simulink model "LQR_Controller"  (R2023b)
settings: Solver=VariableStepAuto  StartTime=0.0  StopTime=100  RelTol=1e-3
values from neighbouring files (symbols this model uses):
  k1 = K(3,1)    [LQR.m]
  k10 = K(3,10)    [LQR.m]
  k11 = K(4,11)    [LQR.m]
  k12 = K(4,12)    [LQR.m]
  k2 = K(3,2)    [LQR.m]
  k3 = K(2,3)    [LQR.m]
  k5 = K(1,5)    [LQR.m]
  k6 = K(1,6)    [LQR.m]
  k7 = K(2,7)    [LQR.m]
  k8 = K(2,8)    [LQR.m]
  k9 = K(3,9)    [LQR.m]
  ki13 = Ki(3,13)    [LQR.m]
  ki14 = Ki(2,14)    [LQR.m]
undefined symbols (not defined in the file or in its folder): g, m
settings Model: Creator=DELL  LastModifiedBy=DELL

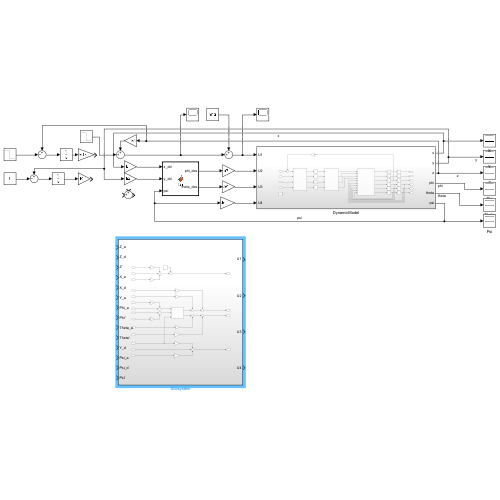
[thumbnail: Simulink's stored preview of the top-level diagram]
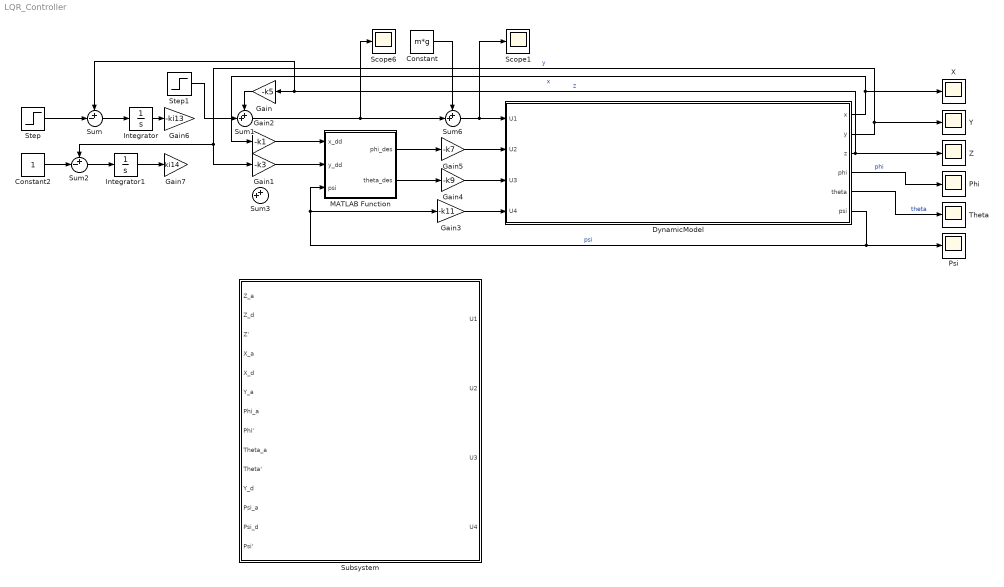
== system LQR_Controller ==
  Constant : Constant  Value=m*g
  Constant2 : Constant
  DynamicModel : Subsystem
  Gain : Gain  Gain=-k5
  Gain1 : Gain  Gain=-k3
  Gain2 : Gain  Gain=-k1
  Gain3 : Gain  Gain=-k11
  Gain4 : Gain  Gain=-k9
  Gain5 : Gain  Gain=-k7
  Gain6 : Gain  Gain=-ki13
  Gain7 : Gain  Gain=ki14
  Integrator : Integrator
  Integrator1 : Integrator
  MATLAB Function : MATLAB Function  TreatAsAtomicUnit=on
  Phi : Scope
  Psi : Scope
  Scope1 : Scope
  Scope6 : Scope
  Step : Step  After=-1  SampleTime=0
  Step1 : Step  After=-1  SampleTime=0
  Subsystem : Subsystem
  Sum : Sum  Inputs=+-|
  Sum1 : Sum  Inputs=++|
  Sum2 : Sum  Inputs=+-|
  Sum3 : Sum  Inputs=++|
  Sum6 : Sum  Inputs=++|
  Theta : Scope
  X : Scope
  Y : Scope
  Z : Scope
  wires:
  DynamicModel/3(z) -> Z/1, Sum/1, Gain/1  "z"
  DynamicModel/2(y) -> Y/1, Sum2/1, Gain1/1  "y"
  DynamicModel/1(x) -> Gain2/1, X/1  "x"
  DynamicModel/6(psi) -> Psi/1, Gain3/1, MATLAB Function/3(psi)  "psi"
  DynamicModel/4(phi) -> Phi/1  "phi"
  DynamicModel/5(theta) -> Theta/1  "theta"
  MATLAB Function/2(theta_des) -> Gain4/1
  Gain2/1 -> MATLAB Function/1(x_dd)
  Gain3/1 -> DynamicModel/4(U4)
  MATLAB Function/1(phi_des) -> Gain5/1
  Gain5/1 -> DynamicModel/2(U2)
  Gain4/1 -> DynamicModel/3(U3)
  Sum6/1 -> Scope1/1, DynamicModel/1(U1)
  Constant/1 -> Sum6/1
  Step/1 -> Sum/2
  Sum/1 -> Integrator/1
  Integrator/1 -> Gain6/1
  Gain/1 -> Sum1/1
  Sum1/1 -> Sum6/2, Scope6/1
  Integrator1/1 -> Gain7/1
  Sum2/1 -> Integrator1/1
  Constant2/1 -> Sum2/2
  Step1/1 -> Sum1/2
  Gain1/1 -> MATLAB Function/2(y_dd)

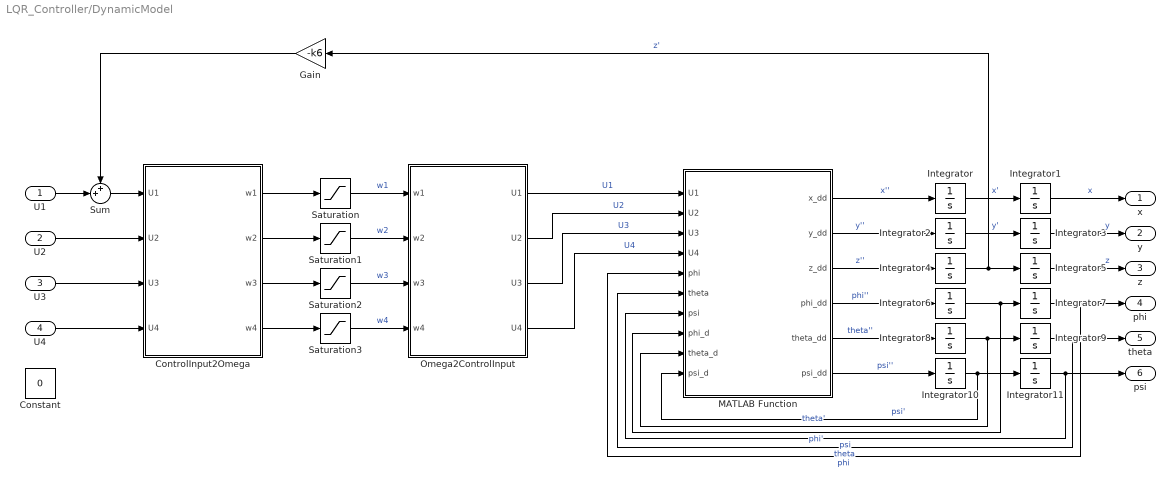
== system LQR_Controller/DynamicModel ==
  U1 : Inport
  U2 : Inport  Port=2
  U3 : Inport  Port=3
  U4 : Inport  Port=4
  Constant : Constant  Value=0
  ControlInput2Omega : MATLAB Function  TreatAsAtomicUnit=on
  Gain : Gain  Gain=-k6
  Integrator{,1..11} (12 alike) : Integrator
  MATLAB Function : MATLAB Function  TreatAsAtomicUnit=on
  Omega2ControlInput : MATLAB Function  TreatAsAtomicUnit=on
  Saturation{,1..3} (4 alike) : Saturate  UpperLimit=550  LowerLimit=0
  Sum : Sum  Inputs=++|
  x : Outport
  y : Outport  Port=2
  z : Outport  Port=3
  phi : Outport  Port=4
  theta : Outport  Port=5
  psi : Outport  Port=6
  wires:
  Integrator8/1 -> MATLAB Function/9(theta_d), Integrator9/1  "theta'"
  ControlInput2Omega/3(w3) -> Saturation2/1
  Integrator5/1 -> z/1  "z"
  MATLAB Function/1(x_dd) -> Integrator/1  "x''"
  MATLAB Function/5(theta_dd) -> Integrator8/1  "theta''"
  MATLAB Function/6(psi_dd) -> Integrator10/1  "psi''"
  MATLAB Function/3(z_dd) -> Integrator4/1  "z''"
  Saturation2/1 -> Omega2ControlInput/3(w3)  "w3"
  Integrator10/1 -> MATLAB Function/10(psi_d), Integrator11/1  "psi'"
  Integrator6/1 -> MATLAB Function/8(phi_d), Integrator7/1  "phi'"
  MATLAB Function/4(phi_dd) -> Integrator6/1  "phi''"
  Integrator3/1 -> y/1  "y"
  Saturation1/1 -> Omega2ControlInput/2(w2)  "w2"
  ControlInput2Omega/4(w4) -> Saturation3/1
  Integrator4/1 -> Gain/1, Integrator5/1  "z'"
  Saturation/1 -> Omega2ControlInput/1(w1)  "w1"
  Saturation3/1 -> Omega2ControlInput/4(w4)  "w4"
  Integrator11/1 -> psi/1, MATLAB Function/7(psi)  "psi"
  MATLAB Function/2(y_dd) -> Integrator2/1  "y''"
  Integrator2/1 -> Integrator3/1  "y'"
  Integrator7/1 -> phi/1, MATLAB Function/5(phi)  "phi"
  Integrator1/1 -> x/1  "x"
  Integrator/1 -> Integrator1/1  "x'"
  ControlInput2Omega/2(w2) -> Saturation1/1
  Integrator9/1 -> theta/1, MATLAB Function/6(theta)  "theta"
  ControlInput2Omega/1(w1) -> Saturation/1
  Omega2ControlInput/1(U1) -> MATLAB Function/1(U1)  "U1"
  Omega2ControlInput/2(U2) -> MATLAB Function/2(U2)  "U2"
  Omega2ControlInput/3(U3) -> MATLAB Function/3(U3)  "U3"
  Omega2ControlInput/4(U4) -> MATLAB Function/4(U4)  "U4"
  U4/1 -> ControlInput2Omega/4(U4)
  U3/1 -> ControlInput2Omega/3(U3)
  U2/1 -> ControlInput2Omega/2(U2)
  U1/1 -> Sum/2
  Sum/1 -> ControlInput2Omega/1(U1)
  Gain/1 -> Sum/1

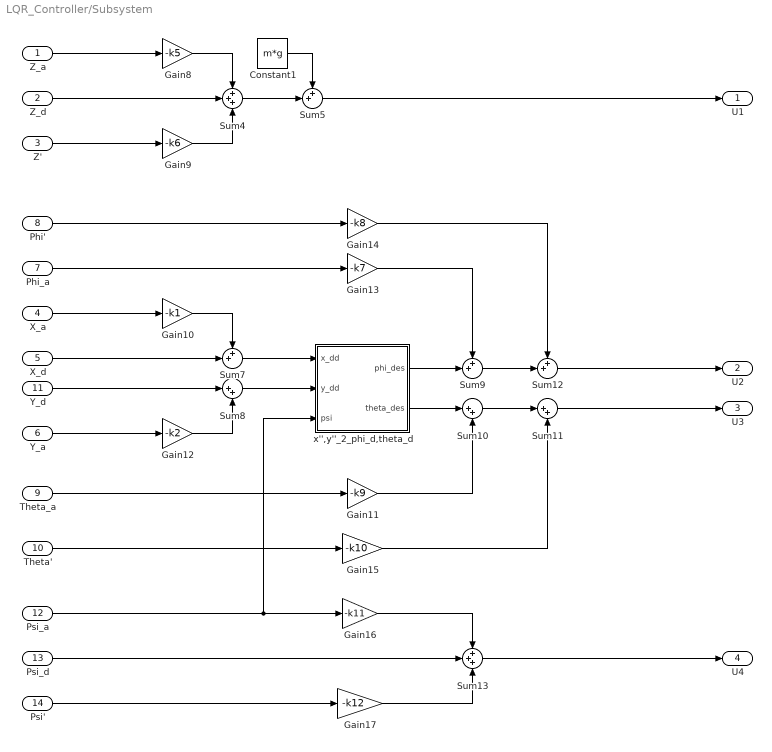
== system LQR_Controller/Subsystem ==
  Z_a : Inport
  Z_d : Inport  Port=2
  Z' : Inport  Port=3
  X_a : Inport  Port=4
  X_d : Inport  Port=5
  Y_a : Inport  Port=6
  Phi_a : Inport  Port=7
  Phi' : Inport  Port=8
  Theta_a : Inport  Port=9
  Theta' : Inport  Port=10
  Y_d : Inport  Port=11
  Psi_a : Inport  Port=12
  Psi_d : Inport  Port=13
  Psi' : Inport  Port=14
  Constant1 : Constant  Value=m*g
  Gain10 : Gain  Gain=-k1
  Gain11 : Gain  Gain=-k9
  Gain12 : Gain  Gain=-k2
  Gain13 : Gain  Gain=-k7
  Gain14 : Gain  Gain=-k8
  Gain15 : Gain  Gain=-k10
  Gain16 : Gain  Gain=-k11
  Gain17 : Gain  Gain=-k12
  Gain8 : Gain  Gain=-k5
  Gain9 : Gain  Gain=-k6
  Sum10 : Sum  Inputs=|++
  Sum11 : Sum  Inputs=|++
  Sum{5,7,9,12} (4 alike) : Sum  Inputs=++|
  Sum13 : Sum  Inputs=+++
  Sum4 : Sum  Inputs=+++
  Sum8 : Sum  Inputs=|++
  x'',y''_2_phi_d,theta_d : MATLAB Function  TreatAsAtomicUnit=on
  U1 : Outport
  U2 : Outport  Port=2
  U3 : Outport  Port=3
  U4 : Outport  Port=4
  wires:
  Theta_a/1 -> Gain11/1
  Gain8/1 -> Sum4/1
  x'',y''_2_phi_d,theta_d/2(theta_des) -> Sum10/1
  X_a/1 -> Gain10/1
  Y_a/1 -> Gain12/1
  Sum12/1 -> U2/1
  Z'/1 -> Gain9/1
  Gain17/1 -> Sum13/3
  Sum13/1 -> U4/1
  X_d/1 -> Sum7/2
  Sum8/1 -> x'',y''_2_phi_d,theta_d/2(y_dd)
  Sum4/1 -> Sum5/2
  Psi'/1 -> Gain17/1
  Z_a/1 -> Gain8/1
  Sum9/1 -> Sum12/2
  Gain9/1 -> Sum4/3
  Phi'/1 -> Gain14/1
  Gain16/1 -> Sum13/1
  Gain15/1 -> Sum11/2
  Y_d/1 -> Sum8/1
  Constant1/1 -> Sum5/1
  Gain13/1 -> Sum9/1
  Phi_a/1 -> Gain13/1
  Gain10/1 -> Sum7/1
  x'',y''_2_phi_d,theta_d/1(phi_des) -> Sum9/2
  Sum7/1 -> x'',y''_2_phi_d,theta_d/1(x_dd)
  Gain12/1 -> Sum8/2
  Gain14/1 -> Sum12/1
  Gain11/1 -> Sum10/2
  Psi_d/1 -> Sum13/2
  Sum10/1 -> Sum11/1
  Psi_a/1 -> x'',y''_2_phi_d,theta_d/3(psi), Gain16/1
  Sum11/1 -> U3/1
  Sum5/1 -> U1/1
  Theta'/1 -> Gain15/1
  Z_d/1 -> Sum4/2

== matlab function LQR_Controller/DynamicModel/Omega2ControlInput ==
  data: w1 input; U1 output; w2 input; w3 input; w4 input; U2 output; U3 output; U4 output
function [U1,U2,U3,U4] = fcn(w1,w2,w3,w4)
    
    % COEFFITIENTS
    Kf = 3.13e-5;
    Km = 7.5e-7;

    U1 = Kf * ((w1^2)+(w2^2)+(w3^2)+(w4^2));
    U2 = Kf * (-(w2^2)+(w4^2));
    U3 = Kf * ((w1^2)-(w3^2));
    U4 = Km * ((w1^2)-(w2^2)+(w3^2)-(w4^2));

== matlab function LQR_Controller/DynamicModel/MATLAB Function ==
  data: U1 input; x_dd output; U2 input; U3 input; U4 input; phi input; theta input; psi input; phi_d input; theta_d input; psi_d input; y_dd output; z_dd output; phi_dd output; theta_dd output; psi_dd output
function [x_dd,y_dd,z_dd,phi_dd,theta_dd,psi_dd] = fcn(U1,U2,U3,U4, phi,theta,psi, phi_d, theta_d, psi_d)
    
    % MOMENTS OF INERTIA
    Ixx = 7.5e-3;
    Iyy = 7.5e-3;
    Izz = 1.3e-2;
    
    % GYRO
    Jr = 0;
    wr = 0;
    
    % LENGTH
    l = 0.23;
    
    % MASS & GRAVITATIONAL ACCELERATION
    m = 0.65;
    g = 9.81;
    
    x_dd = -(U1/m)*(sin(phi)*sin(psi)+cos(phi)*cos(psi)*sin(theta));
    y_dd = -(U1/m)*(cos(phi)*sin(psi)*sin(theta)-cos(psi)*sin(phi));
    z_dd = g - (U1/m)*(cos(phi)*cos(theta));

    phi_dd = (l/Ixx)*U2 - (Jr/Ixx)*theta_d*wr + (Iyy/Ixx)*psi_d*theta_d - (Izz/Ixx)*theta_d*psi_d;
    theta_dd = (l/Iyy)*U3 - (Jr/Iyy)*phi_d*wr + (Izz/Iyy)*phi_d*psi_d - (Ixx/Iyy)*psi_d*phi_d;
    psi_dd = (1/Izz)*U4 + (Ixx/Izz)*theta_d*phi_d - (Iyy/Izz)*phi_d*theta_d;

y = [x_dd,y_dd,z_dd,phi_dd,theta_dd,psi_dd];

== matlab function LQR_Controller/DynamicModel/ControlInput2Omega ==
  data: U1 input; w1 output; U2 input; U3 input; U4 input; w2 output; w3 output; w4 output
function [w1,w2,w3,w4] = fcn(U1,U2,U3,U4)

    % COEFFITIENTS
    Kf = 3.13e-5;
    Km = 7.5e-7;

    w1 = abs((((U1/4)+(U3/2))/Kf + U4/(4*Km)))^(1/2);
    w2 = abs((((U1/4)-(U2/2))/Kf - U4/(4*Km)))^(1/2);
    w3 = abs((((U1/4)-(U3/2))/Kf + U4/(4*Km)))^(1/2);
    w4 = abs((((U1/4)+(U2/2))/Kf - U4/(4*Km)))^(1/2);

    % w1 = sqrt(abs((U1/(4*Kf))+(U3/(2*Kf))+(U4/(4*Km))));
    % w2 = sqrt(abs((U1/(4*Kf))-(U2/(2*Kf))-(U4/(4*Km))));
    % w3 = sqrt(abs((U1/(4*Kf))-(U3/(2*Kf))-(U4/(4*Km))));
    % w4 = sqrt(abs((U1/(4*Kf))+(U2/(2*Kf))-(U4/(4*Km))));

== matlab function LQR_Controller/MATLAB Function ==
  data: x_dd input; phi_des output; y_dd input; psi input; theta_des output
function [phi_des,theta_des] = fcn(x_dd,y_dd,psi)

    g = [-sin(psi) cos(psi); -cos(psi) -sin(psi)]*[x_dd;y_dd];

    phi_des = g(1);
    theta_des = g(2);

== matlab function LQR_Controller/Subsystem/x'',y''_2_phi_d,theta_d ==
  data: x_dd input; phi_des output; y_dd input; psi input; theta_des output
function [phi_des,theta_des] = fcn(x_dd,y_dd,psi)

    g = [-sin(psi) cos(psi); -cos(psi) -sin(psi)]*[x_dd;y_dd];

    phi_des = g(1);
    theta_des = g(2);
